simulink model "barrel_switcher_blk"  (R2019a)
settings: Solver=VariableStepAuto  StartTime=0.0  StopTime=50.0  RelTol=1e-3
libraries: xbsIndex_r4 x61, simulink x2
settings Model: Creator=Ross Donnachie  LastModifiedBy=Ross Donnachie

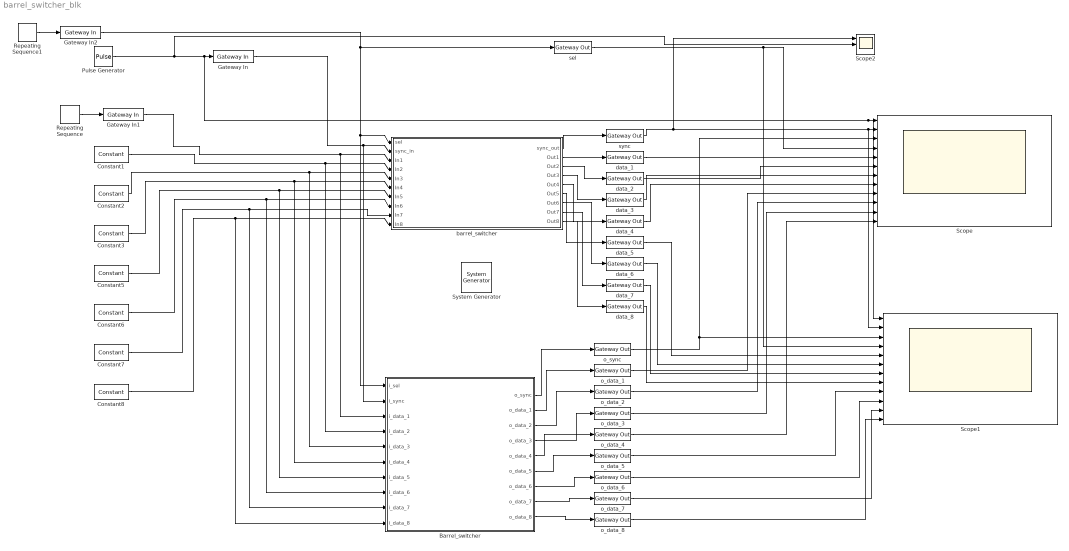
== system barrel_switcher_blk ==
  " System Generator" : xbsIndex_r4/ System Generator  Tag=genX  xilinxfamily=kintex7  part=xc7k325t  speed=-3  package=fbg676  synthesis_tool=Vivado  clock_wrapper=Clock Enables  directory=./netlist  proj_type=Vivado  Synth_file=Vivado Synthesis Defaults  Impl_file=Vivado Implementation Defaults  testbench=off  simulink_period=1  sysclk_period=10  dcm_input_clock_period=10  incr_netlist=off  trim_vbits=Everywhere in SubSystem  dbl_ovrd=According to Block Masks  core_generation=According to Block Masks  run_coregen=off  deprecated_control=off  eval_field=0  block_type=sysgen
  Barrel_switcher : Subsystem  mask{number_of_ports_2exp=3, port_bit_width=4, async=on}
      mask prompts: number_of_ports_2exp "Number of inputs (2^?):"; port_bit_width "Port bit-width:"; async "Asynchronous operation"
      mask init:
      | Simulink.Block.eval([gcb, '/barrel_switcher']);
      | 
      | knit_subsystem_to_blackbox('barrel_switcher');
  Constant1 : xbsIndex_r4/Constant  const=2  gui_display_data_type=Fixed-point  arith_type=Unsigned  n_bits=4  bin_pt=0  preci_type=Single  exp_width=8  frac_width=24  explicit_period=on  period=1  equ=P=C  opselect=C  inp2=PCIN>>17  opr=+  inp1=P  carry=CIN  dbl_ovrd=off  block_type=constant
  Constant2 : xbsIndex_r4/Constant  const=3  gui_display_data_type=Fixed-point  arith_type=Unsigned  n_bits=4  bin_pt=0  preci_type=Single  exp_width=8  frac_width=24  explicit_period=on  period=1  equ=P=C  opselect=C  inp2=PCIN>>17  opr=+  inp1=P  carry=CIN  dbl_ovrd=off  block_type=constant
  Constant3 : xbsIndex_r4/Constant  const=4  gui_display_data_type=Fixed-point  arith_type=Unsigned  n_bits=4  bin_pt=0  preci_type=Single  exp_width=8  frac_width=24  explicit_period=on  period=1  equ=P=C  opselect=C  inp2=PCIN>>17  opr=+  inp1=P  carry=CIN  dbl_ovrd=off  block_type=constant
  Constant5 : xbsIndex_r4/Constant  const=5  gui_display_data_type=Fixed-point  arith_type=Unsigned  n_bits=4  bin_pt=0  preci_type=Single  exp_width=8  frac_width=24  explicit_period=on  period=1  equ=P=C  opselect=C  inp2=PCIN>>17  opr=+  inp1=P  carry=CIN  dbl_ovrd=off  block_type=constant
  Constant6 : xbsIndex_r4/Constant  const=6  gui_display_data_type=Fixed-point  arith_type=Unsigned  n_bits=4  bin_pt=0  preci_type=Single  exp_width=8  frac_width=24  explicit_period=on  period=1  equ=P=C  opselect=C  inp2=PCIN>>17  opr=+  inp1=P  carry=CIN  dbl_ovrd=off  block_type=constant
  Constant7 : xbsIndex_r4/Constant  const=7  gui_display_data_type=Fixed-point  arith_type=Unsigned  n_bits=4  bin_pt=0  preci_type=Single  exp_width=8  frac_width=24  explicit_period=on  period=1  equ=P=C  opselect=C  inp2=PCIN>>17  opr=+  inp1=P  carry=CIN  dbl_ovrd=off  block_type=constant
  Constant8 : xbsIndex_r4/Constant  const=8  gui_display_data_type=Fixed-point  arith_type=Unsigned  n_bits=4  bin_pt=0  preci_type=Single  exp_width=8  frac_width=24  explicit_period=on  period=1  equ=P=C  opselect=C  inp2=PCIN>>17  opr=+  inp1=P  carry=CIN  dbl_ovrd=off  block_type=constant
  Gateway In : xbsIndex_r4/Gateway In  gui_display_data_type=Fixed-point  arith_type=Unsigned  n_bits=1  bin_pt=0  preci_type=Single  exp_width=8  frac_width=24  rows=1  columns=1  quantization="Round  (unbiased: +/- Inf)"  overflow=Saturate  period=1  UseAsADC=off  ADCChannel='1'  interface=None  automatic_assignment=on  address_offset=hex2dec('00')  intf_name=''  intf_description=''  default_value=0  timing_constraint=None  locs_specified=off  LOCs={}  io_standard={}  inherit_from_input=off  hdl_port=on  dbl_ovrd=off  block_type=gatewayin
  Gateway In1 : xbsIndex_r4/Gateway In  gui_display_data_type=Fixed-point  arith_type=Unsigned  n_bits=4  bin_pt=0  preci_type=Single  exp_width=8  frac_width=24  rows=1  columns=1  quantization="Round  (unbiased: +/- Inf)"  overflow=Saturate  period=1  UseAsADC=off  ADCChannel='1'  interface=None  automatic_assignment=on  address_offset=hex2dec('00')  intf_name=''  intf_description=''  default_value=0  timing_constraint=None  locs_specified=off  LOCs={}  io_standard={}  inherit_from_input=off  hdl_port=on  dbl_ovrd=off  block_type=gatewayin
  Gateway In2 : xbsIndex_r4/Gateway In  gui_display_data_type=Fixed-point  arith_type=Unsigned  n_bits=3  bin_pt=0  preci_type=Single  exp_width=8  frac_width=24  rows=1  columns=1  quantization="Round  (unbiased: +/- Inf)"  overflow=Saturate  period=1  UseAsADC=off  ADCChannel='1'  interface=None  automatic_assignment=on  address_offset=hex2dec('00')  intf_name=''  intf_description=''  default_value=0  timing_constraint=None  locs_specified=off  LOCs={}  io_standard={}  inherit_from_input=off  hdl_port=on  dbl_ovrd=off  block_type=gatewayin
  Pulse Generator : DiscretePulseGenerator  PulseType=Time based  Period=20  PulseWidth=50  PhaseDelay=2
  Repeating Sequence : simulink/Sources/Repeating Sequence  rep_seq_t=[0 22]  rep_seq_y=[1 5]
  Repeating Sequence1 : simulink/Sources/Repeating Sequence  rep_seq_t=[0 50]  rep_seq_y=[2 2]
  Scope : Scope  NumInputPorts=12
  Scope1 : Scope  NumInputPorts=12
  Scope2 : Scope  NumInputPorts=3
  barrel_switcher : Subsystem  AncestorBlock=casper_library_reorder/barrel_switcher  mask(barrel_switcher){n_inputs=3, async=off}
      mask prompts: n_inputs "Number of Inputs: (2^?)"; async "Asynchronous operation"
      mask help:
      | Shifts input to right by amount specified on sel,
      | wrapping around into higher order bits.
      mask init:
      | barrel_switcher_init(gcb,...
      |     'n_inputs', n_inputs, ...
      |     'async', async);
      mask Help: eval('xlWeb(''http://casper.berkeley.edu/wiki/Barrel_switcher'')')
  data_{1..8} (8 alike) : xbsIndex_r4/Gateway Out  inherit_from_input=on  hdl_port=on  rows=1  columns=1  UseAsDAC=off  DACChannel='1'  interface=None  automatic_assignment=on  address_offset=hex2dec('00')  intf_name=''  intf_description=''  timing_constraint=None  locs_specified=off  LOCs={}  io_standard={}  block_type=gatewayout
  o_data_{1..8} (8 alike) : xbsIndex_r4/Gateway Out  inherit_from_input=on  hdl_port=on  rows=1  columns=1  UseAsDAC=off  DACChannel='1'  interface=None  automatic_assignment=on  address_offset=hex2dec('00')  intf_name=''  intf_description=''  timing_constraint=None  locs_specified=off  LOCs={}  io_standard={}  block_type=gatewayout
  o_sync : xbsIndex_r4/Gateway Out  inherit_from_input=on  hdl_port=on  rows=1  columns=1  UseAsDAC=off  DACChannel='1'  interface=None  automatic_assignment=on  address_offset=hex2dec('00')  intf_name=''  intf_description=''  timing_constraint=None  locs_specified=off  LOCs={}  io_standard={}  block_type=gatewayout
  sel : xbsIndex_r4/Gateway Out  inherit_from_input=on  hdl_port=on  rows=1  columns=1  UseAsDAC=off  DACChannel='1'  interface=None  automatic_assignment=on  address_offset=hex2dec('00')  intf_name=''  intf_description=''  timing_constraint=None  locs_specified=off  LOCs={}  io_standard={}  block_type=gatewayout
  sync : xbsIndex_r4/Gateway Out  inherit_from_input=on  hdl_port=on  rows=1  columns=1  UseAsDAC=off  DACChannel='1'  interface=None  automatic_assignment=on  address_offset=hex2dec('00')  intf_name=''  intf_description=''  timing_constraint=None  locs_specified=off  LOCs={}  io_standard={}  block_type=gatewayout
  wires:
  Constant2/1 -> Barrel_switcher/5(i_data_3), barrel_switcher/5(In3)
  Gateway In2/1 -> Barrel_switcher/1(i_sel), barrel_switcher/1(sel), sel/1
  Pulse Generator/1 -> Scope2/2, Scope1/1, Scope/1, Gateway In/1
  Constant1/1 -> Barrel_switcher/4(i_data_2), barrel_switcher/4(In2)
  Gateway In/1 -> Barrel_switcher/2(i_sync), barrel_switcher/2(sync_in)
  barrel_switcher/1(sync_out) -> sync/1
  barrel_switcher/2(Out1) -> data_1/1
  barrel_switcher/3(Out2) -> data_2/1
  barrel_switcher/4(Out3) -> data_3/1
  barrel_switcher/5(Out4) -> data_4/1
  sync/1 -> Scope2/1, Scope1/2, Scope/2
  o_sync/1 -> Scope1/3, Scope/3
  data_1/1 -> Scope/5
  data_2/1 -> Scope/6
  data_3/1 -> Scope/7
  data_4/1 -> Scope/8
  o_data_1/1 -> Scope/9
  o_data_2/1 -> Scope/10
  o_data_3/1 -> Scope/11
  o_data_4/1 -> Scope/12
  Repeating Sequence/1 -> Gateway In1/1
  Constant3/1 -> Barrel_switcher/6(i_data_4), barrel_switcher/6(In4)
  Constant5/1 -> Barrel_switcher/7(i_data_5), barrel_switcher/7(In5)
  Constant6/1 -> Barrel_switcher/8(i_data_6), barrel_switcher/8(In6)
  Constant7/1 -> Barrel_switcher/9(i_data_7), barrel_switcher/9(In7)
  Constant8/1 -> Barrel_switcher/10(i_data_8), barrel_switcher/10(In8)
  barrel_switcher/6(Out5) -> data_5/1
  barrel_switcher/7(Out6) -> data_6/1
  barrel_switcher/8(Out7) -> data_7/1
  barrel_switcher/9(Out8) -> data_8/1
  data_5/1 -> Scope1/5
  data_6/1 -> Scope1/6
  data_7/1 -> Scope1/7
  data_8/1 -> Scope1/8
  o_data_5/1 -> Scope1/9
  o_data_6/1 -> Scope1/10
  o_data_7/1 -> Scope1/11
  o_data_8/1 -> Scope1/12
  Gateway In1/1 -> Barrel_switcher/3(i_data_1), barrel_switcher/3(In1)
  Repeating Sequence1/1 -> Gateway In2/1
  sel/1 -> Scope1/4, Scope/4
  Barrel_switcher/1(o_sync) -> o_sync/1
  Barrel_switcher/2(o_data_1) -> o_data_1/1
  Barrel_switcher/3(o_data_2) -> o_data_2/1
  Barrel_switcher/4(o_data_3) -> o_data_3/1
  Barrel_switcher/5(o_data_4) -> o_data_4/1
  Barrel_switcher/6(o_data_5) -> o_data_5/1
  Barrel_switcher/7(o_data_6) -> o_data_6/1
  Barrel_switcher/8(o_data_7) -> o_data_7/1
  Barrel_switcher/9(o_data_8) -> o_data_8/1

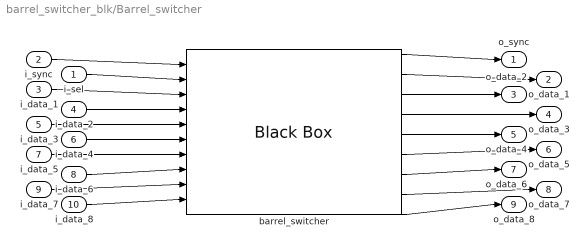
== system barrel_switcher_blk/Barrel_switcher ==
  i_sel : Inport
  i_sync : Inport  Port=2
  i_data_1 : Inport  Port=3
  i_data_2 : Inport  Port=4
  i_data_3 : Inport  Port=5
  i_data_4 : Inport  Port=6
  i_data_5 : Inport  Port=7
  i_data_6 : Inport  Port=8
  i_data_7 : Inport  Port=9
  i_data_8 : Inport  Port=10
  barrel_switcher : xbsIndex_r4/Black Box  init_code=barrel_switcher_config  sim_method=ISE Simulator  verbose=on  block_type=blackbox2
  o_sync : Outport
  o_data_1 : Outport  Port=2
  o_data_2 : Outport  Port=3
  o_data_3 : Outport  Port=4
  o_data_4 : Outport  Port=5
  o_data_5 : Outport  Port=6
  o_data_6 : Outport  Port=7
  o_data_7 : Outport  Port=8
  o_data_8 : Outport  Port=9
  wires:
  i_sync/1 -> barrel_switcher/1
  i_sel/1 -> barrel_switcher/2
  i_data_1/1 -> barrel_switcher/3
  i_data_2/1 -> barrel_switcher/4
  i_data_3/1 -> barrel_switcher/5
  i_data_4/1 -> barrel_switcher/6
  i_data_5/1 -> barrel_switcher/7
  i_data_6/1 -> barrel_switcher/8
  i_data_7/1 -> barrel_switcher/9
  i_data_8/1 -> barrel_switcher/10
  barrel_switcher/1 -> o_sync/1
  barrel_switcher/2 -> o_data_1/1
  barrel_switcher/3 -> o_data_2/1
  barrel_switcher/4 -> o_data_3/1
  barrel_switcher/5 -> o_data_4/1
  barrel_switcher/6 -> o_data_5/1
  barrel_switcher/7 -> o_data_6/1
  barrel_switcher/8 -> o_data_7/1
  barrel_switcher/9 -> o_data_8/1

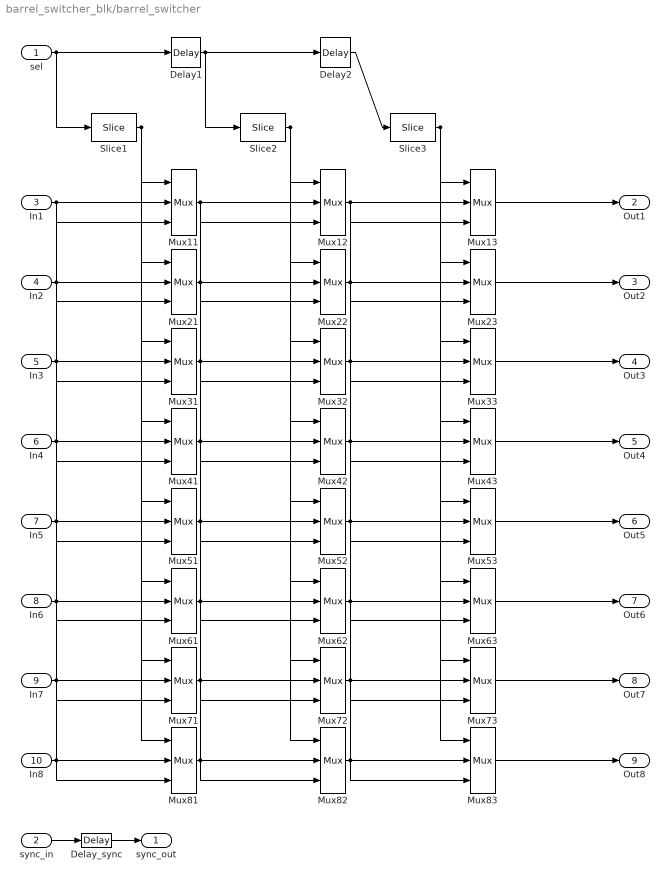
== system barrel_switcher_blk/barrel_switcher ==
  sel : Inport
  sync_in : Inport  Port=2
  In1 : Inport  Port=3
  In2 : Inport  Port=4
  In3 : Inport  Port=5
  In4 : Inport  Port=6
  In5 : Inport  Port=7
  In6 : Inport  Port=8
  In7 : Inport  Port=9
  In8 : Inport  Port=10
  Delay1 : xbsIndex_r4/Delay  rst=off  infoeditControl=Selection of Reset will increase slice count due to use of real FFs and instead of SRLs  en=off  latency=1  reg_retiming=on  dbl_ovrd=off  block_type=delay
  Delay2 : xbsIndex_r4/Delay  rst=off  infoeditControl=Selection of Reset will increase slice count due to use of real FFs and instead of SRLs  en=off  latency=1  reg_retiming=on  dbl_ovrd=off  block_type=delay
  Delay_sync : xbsIndex_r4/Delay  rst=off  infoeditControl=Selection of Reset will increase slice count due to use of real FFs and instead of SRLs  en=off  latency=3  reg_retiming=on  dbl_ovrd=off  block_type=delay
  Mux{11..13,21..23,31..33,41..43,51..53,61..63,71..73,81..83} (24 alike) : xbsIndex_r4/Mux  inputs=2  en=off  latency=1  precision=Full  arith_type=Unsigned  n_bits=16  bin_pt=14  quantization=Truncate  overflow=Wrap  dbl_ovrd=off  block_type=mux
  Slice1 : xbsIndex_r4/Slice  nbits=1  boolean_output=off  mode=Upper Bit Location + Width  bit1=-0  base1=MSB of Input  bit0=0  base0=LSB of Input  dbl_ovrd=off  block_type=slice
  Slice2 : xbsIndex_r4/Slice  nbits=1  boolean_output=off  mode=Upper Bit Location + Width  bit1=-1  base1=MSB of Input  bit0=0  base0=LSB of Input  dbl_ovrd=off  block_type=slice
  Slice3 : xbsIndex_r4/Slice  nbits=1  boolean_output=off  mode=Upper Bit Location + Width  bit1=-2  base1=MSB of Input  bit0=0  base0=LSB of Input  dbl_ovrd=off  block_type=slice
  sync_out : Outport
  Out1 : Outport  Port=2
  Out2 : Outport  Port=3
  Out3 : Outport  Port=4
  Out4 : Outport  Port=5
  Out5 : Outport  Port=6
  Out6 : Outport  Port=7
  Out7 : Outport  Port=8
  Out8 : Outport  Port=9
  wires:
  sync_in/1 -> Delay_sync/1
  Delay_sync/1 -> sync_out/1
  sel/1 -> Slice1/1, Delay1/1
  Delay1/1 -> Delay2/1, Slice2/1
  Delay2/1 -> Slice3/1
  Slice1/1 -> Mux11/1, Mux21/1, Mux31/1, Mux41/1, Mux51/1, Mux61/1, Mux71/1, Mux81/1
  Slice2/1 -> Mux12/1, Mux22/1, Mux32/1, Mux42/1, Mux52/1, Mux62/1, Mux72/1, Mux82/1
  Slice3/1 -> Mux13/1, Mux23/1, Mux33/1, Mux43/1, Mux53/1, Mux63/1, Mux73/1, Mux83/1
  In1/1 -> Mux11/2, Mux51/3
  Mux13/1 -> Out1/1
  In2/1 -> Mux21/2, Mux61/3
  Mux23/1 -> Out2/1
  In3/1 -> Mux31/2, Mux71/3
  Mux33/1 -> Out3/1
  In4/1 -> Mux41/2, Mux81/3
  Mux43/1 -> Out4/1
  In5/1 -> Mux51/2, Mux11/3
  Mux53/1 -> Out5/1
  In6/1 -> Mux61/2, Mux21/3
  Mux63/1 -> Out6/1
  In7/1 -> Mux71/2, Mux31/3
  Mux73/1 -> Out7/1
  In8/1 -> Mux81/2, Mux41/3
  Mux83/1 -> Out8/1
  Mux11/1 -> Mux12/2, Mux72/3
  Mux12/1 -> Mux13/2, Mux83/3
  Mux21/1 -> Mux22/2, Mux82/3
  Mux22/1 -> Mux23/2, Mux13/3
  Mux31/1 -> Mux32/2, Mux12/3
  Mux32/1 -> Mux33/2, Mux23/3
  Mux41/1 -> Mux42/2, Mux22/3
  Mux42/1 -> Mux43/2, Mux33/3
  Mux51/1 -> Mux52/2, Mux32/3
  Mux52/1 -> Mux53/2, Mux43/3
  Mux61/1 -> Mux62/2, Mux42/3
  Mux62/1 -> Mux63/2, Mux53/3
  Mux71/1 -> Mux72/2, Mux52/3
  Mux72/1 -> Mux73/2, Mux63/3
  Mux81/1 -> Mux82/2, Mux62/3
  Mux82/1 -> Mux83/2, Mux73/3
